simulink model "Control_For_exp1"  (R2015b)
settings: Solver=VariableStepAuto  StartTime=0.0  StopTime=10.0  RelTol=1e-3
StartFcn:
  | open_scope
settings Model: Creator=LUBO  LastModifiedBy=LUBO

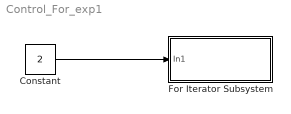
== system Control_For_exp1 ==
  Constant : Constant  Value=2
  For Iterator Subsystem : Subsystem  TreatAsAtomicUnit=on
  wires:
  Constant/1 -> For Iterator Subsystem/1(In1)

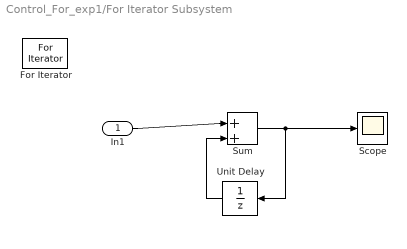
== system Control_For_exp1/For Iterator Subsystem ==
  In1 : Inport
  For Iterator : ForIterator  ShowIterationPort=off
  Scope : Scope
  Sum : Sum  Inputs=|++
  Unit Delay : UnitDelay  SampleTime=-1
  wires:
  In1/1 -> Sum/1
  Sum/1 -> Scope/1, Unit Delay/1
  Unit Delay/1 -> Sum/2
